simulink model "model_1"  (R2014a)
settings: Solver=ode3  StartTime=0.0  StopTime=30  FixedStep=0.1  RelTol=1e-3
libraries: simulink x3
settings Model: Creator=Павел  LastModifiedBy=Павел
settings DataIOCC: InspectSignalLogs=on

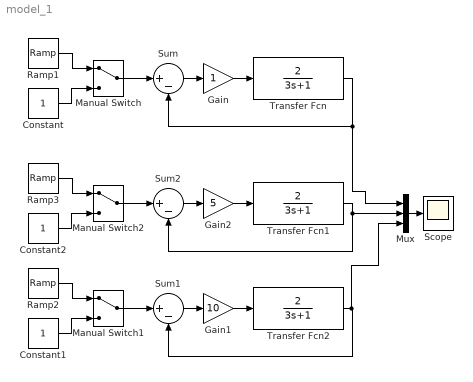
== system model_1 ==
  Constant : Constant
  Constant1 : Constant
  Constant2 : Constant
  Gain : Gain
  Gain1 : Gain  Gain=10
  Gain2 : Gain  Gain=5
  Manual Switch : ManualSwitch
  Manual Switch1 : ManualSwitch
  Manual Switch2 : ManualSwitch
  Mux : Mux  Inputs=3
  Ramp1 : simulink/Sources/Ramp  slope=0.5  start=0  X0=0
  Ramp2 : simulink/Sources/Ramp  slope=0.5  start=0  X0=0
  Ramp3 : simulink/Sources/Ramp  slope=0.5  start=0  X0=0
  Scope : Scope
      settings: TimeRange=30
  Sum : Sum  Inputs=|+-
  Sum1 : Sum  Inputs=|+-
  Sum2 : Sum  Inputs=|+-
  Transfer Fcn : TransferFcn  Numerator=[2]  Denominator=[3 1]
  Transfer Fcn1 : TransferFcn  Numerator=[2]  Denominator=[3 1]
  Transfer Fcn2 : TransferFcn  Numerator=[2]  Denominator=[3 1]
  wires:
  Sum/1 -> Gain/1
  Transfer Fcn/1 -> Mux/1, Sum/2
  Constant/1 -> Manual Switch/2
  Manual Switch/1 -> Sum/1
  Gain/1 -> Transfer Fcn/1
  Ramp1/1 -> Manual Switch/1
  Sum1/1 -> Gain1/1
  Transfer Fcn2/1 -> Mux/3, Sum1/2
  Constant1/1 -> Manual Switch1/2
  Manual Switch1/1 -> Sum1/1
  Gain1/1 -> Transfer Fcn2/1
  Ramp2/1 -> Manual Switch1/1
  Sum2/1 -> Gain2/1
  Transfer Fcn1/1 -> Mux/2, Sum2/2
  Constant2/1 -> Manual Switch2/2
  Manual Switch2/1 -> Sum2/1
  Gain2/1 -> Transfer Fcn1/1
  Ramp3/1 -> Manual Switch2/1
  Mux/1 -> Scope/1
